simulink library "vmc"  (R2021b)
settings: Solver=VariableStepAuto  StartTime=0.0  StopTime=10.0  RelTol=1e-3
undefined symbols (not defined in the file or in its folder): AVMC_ACCDeltaTqIGain_X_kph, AVMC_ACCDeltaTqIGain_Y_mps2, AVMC_ACCDeltaTqIGainP2_X_kph, AVMC_ACCDeltaTqIGainP2_Y_mps2, AVMC_ACCDeltaTqPGain_X_kph, AVMC_ACCDeltaTqPGain_Y_kph, AVMC_ACCDeltaTqPGainP2_X_kph, AVMC_ACCDeltaTqPGainP2_Y_kph, AVMC_ACCLongSteadyCtrl_X_kph, AVMC_CCAccelCMD_X_kph, AVMC_CCAccelCMD_Y_kph, AVMC_CCDeltaTqIGain_X_kph, AVMC_CCDeltaTqIGain_Y_mps2, AVMC_CCDeltaTqPGain_X_kph, AVMC_CCDeltaTqPGain_Y_kph, AVMC_CCLongSteadyCtrl_X_kph, AVMC_DISCDeltaTqIGainP2_X_kph, AVMC_DISCDeltaTqIGainP2_Y_mps2, AVMC_ESCRegenOut_X_kph, AVMC_ESCRegenOut_Y_Deg, AVMC_ESCRegenOutEnSpd_X_Deg, AVMC_LatESCRegenOut_X_kph, AVMC_LatESCRegenOut_Y_Deg, AVMC_LongAccDeadZone_X_kph, AVMC_LongAccDeadZoneP2_X_kph, AVMC_LongAccFiltTs_X_Gps, AVMC_LongAccFiltTsP2_X_Gps, AVMC_MCPresBaseTq_X_bar, AVMC_MSAAccelCMD_X_kph, AVMC_MSAAccelCMD_Y_kph, AVMC_MSADeltaTqIGain_X_kph, AVMC_MSADeltaTqIGain_Y_mps2, AVMC_MSADeltaTqPGain_X_kph, AVMC_MSADeltaTqPGain_Y_kph, AVMC_MSALongSteadyCtrl_X_kph, AVMC_MSAPedalOvrd_X_kph, AVMC_MSASpdBand_X_kph, AVMC_OPDDisSlideRate_X_Deg, AVMC_RDCDetectTime_X_kph, AVMC_RDCDetectTime_Y_pct, AVMC_RDCEnSlideRate_X_Deg, AVMC_StESCYaw_X_kph, AVMC_StESCYaw_Y_Deg, AVMC_StESCYawCom_X_kph, AVMC_StESCYawCom_Y_Gps, AVMC_TMSpdBaseTq_X_rpm, C_TASK_10MS_S, C_TASK_5MS_S, DEG2RAD, Discrete, ENUM_ADASACCSTA_ACTIVE, ENUM_ADASACCSTA_OVERRIDE, ENUM_ADASACCSTA_STANDBY, ENUM_ADASMSASTA_ACTIVE, ENUM_ADASMSASTA_ERROR, ENUM_ADASMSASTA_OFF, ENUM_ADASMSASTA_OVERSPEED, ENUM_ADASMSASTA_STANDBY, ENUM_ADASMSASTA_UNDERSPEED, ENUM_ADASMSASTA_UNLIMIT ... (+254)
libraries: hcu_lib x57, simulink x49, ctrlSharedLib x6, simulink_extras x1
(part 4 of 9)

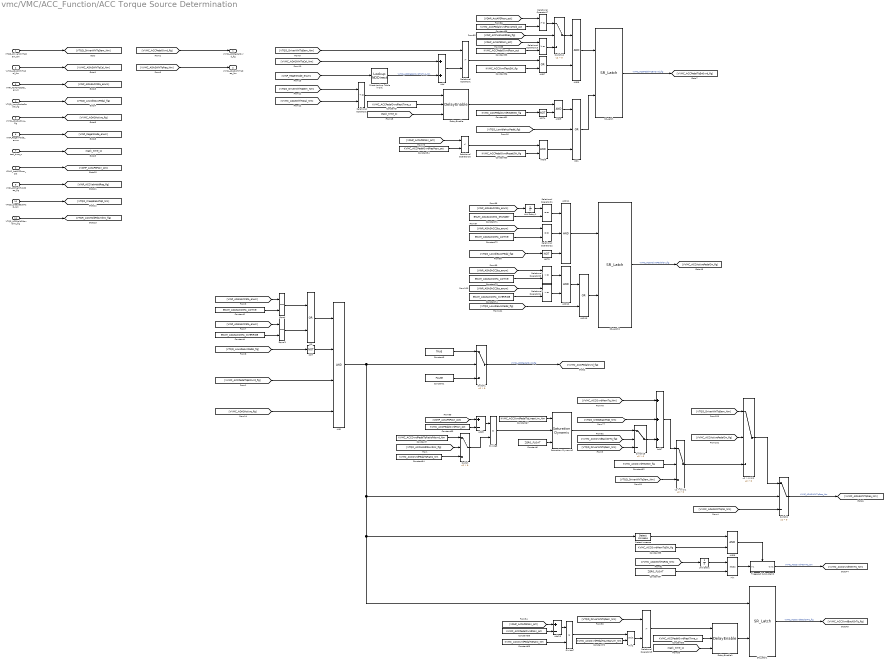
== system vmc/VMC/ACC_Function/ACC Torque Source Determination ==
  VTQD_DriverWhlTqDem_Nm : Inport
  VVMC_ADASWhlTqCal_Nm : Inport  Port=2
  VINP_ADASACCSta_enum : Inport  Port=3
  VTQD_LowIdleAccPedal_flg : Inport  Port=4
  VVMC_ADASActive_flg : Inport  Port=5
  VINP_RegenMode_enum : Inport  Port=6
  task_time_s : Inport  Port=7
  VDHP_ActAPSPosn_pct : Inport  Port=8
  VINP_ACCVehHoldReq_flg : Inport  Port=9
  VTQD_CreepBaseTqD_Nm : Inport  Port=10
  VTQR_ACCHoldPdovrdInc_flg : Inport  Port=11
  AND : Logic  Inputs=4  AllPortsSameDT=off  OutDataTypeStr=boolean
  AND11 : Logic  Inputs=3  AllPortsSameDT=off  OutDataTypeStr=boolean
  AND{5..6,8..9,12} (5 alike) : Logic  AllPortsSameDT=off  OutDataTypeStr=boolean
  AND13 : Logic  Operator=OR  AllPortsSameDT=off  OutDataTypeStr=boolean
  AND7 : Logic  Operator=OR  AllPortsSameDT=off  OutDataTypeStr=boolean
  Add : Sum
  Add13 : Sum  Inputs=+-
  Add7 : Sum  Inputs=+++
  Add8 : Sum  Inputs=+-
  Constant1 : Constant  Value=FALSE
  Constant2 : Constant  Value=ENUM_ADASACCSTA_ACTIVE
  Constant3 : Constant  Value=TRUE
  Constant4 : Constant  Value=ENUM_ADASACCSTA_OVERRIDE
  Constant5 : Constant  Value=KVMC_ACCPedalOvrdRestTime_s
  Constant53 : Constant  Value=KVMC_ACCPedalOvrdPosn_pct
  Constant54 : Constant  Value=KVMC_ACCPedalOvrdResPosn_pct
  Constant55 : Constant  Value=KVMC_ACCOvrdMemTqSW_flg
  Constant56 : Constant  Value=KVMC_ACCOvrdTestSW_flg
  Constant57 : Constant  Value=ZERO_FLOAT
  Constant58 : Constant  Value=KVMC_ACCPedalOvrdPosn4Hold_pct
  Constant6 : Constant  Value=ZERO_FLOAT
  Constant60 : Constant  Value=KVMC_ACCPedalOvrdResetSW_flg
  Constant61 : Constant  Value=KVMC_ACCPedalOvrdResetSW_flg
  Constant62 : Constant  Value=KVMC_ACCOvrdTestSW_flg
  Constant63 : Constant  Value=KVMC_ACCPedalOvrdPosn_pct
  Constant64 : Constant  Value=KVMC_ACCOvrdPedalTqRatio_Nm
  Constant66 : Constant  Value=KVMC_ACCPedalOvrdRestTime_s
  Constant67 : Constant  Value=KVMC_ACCOvrdPedalTqLinearLim_Nm
  Constant68 : Constant  Value=KVMC_ACCPedalOvrdPosn_pct
  Constant69 : Constant  Value=KVMC_ACCOvrdPedalTqRatio_Nm
  Constant7 : Constant  Value=KVMC_ACCOvrdPedalTqRatioPdovrd_Nm
  Constant70 : Constant  Value=KVMC_ACCOvrdPedalTqLinearLim_Nm
  Constant71 : Constant  Value=ENUM_ADASACCSTA_STANDBY
  Constant72 : Constant  Value=ENUM_ADASACCSTA_ACTIVE
  Constant73 : Constant  Value=ENUM_ADASACCSTA_ACTIVE
  Constant74 : Constant  Value=ENUM_ADASACCSTA_OVERRIDE
  DelayEnable : hcu_lib/Basic_Blocks/DelayEnable
  DelayEnable1 : hcu_lib/Basic_Blocks/DelayEnable
  Detect Increase : simulink/Logic and Bit Operations/Detect Increase  vinit=0.0  OutDataTypeStr=boolean
  Direct Lookup Table (n-D)1 : LookupNDDirect  NumberOfTableDimensions=1  Table=MVMC_ACCPedalOvrdTqHys_Y_Nm
  Divide5 : Product  Inputs=**
  Divide7 : Product  Inputs=**
  Equal : RelationalOperator  Operator===  OutDataTypeStr=boolean  RndMeth=Simplest
  Equal1 : RelationalOperator  Operator===  OutDataTypeStr=boolean  RndMeth=Simplest
  Min : MinMax  Function=max  Inputs=2
  Min2 : MinMax  Inputs=2
  NOT : Logic  Operator=NOT  AllPortsSameDT=off  OutDataTypeStr=boolean
  NOT4 : Logic  Operator=NOT  AllPortsSameDT=off  OutDataTypeStr=boolean
  NOT5 : Logic  Operator=NOT  AllPortsSameDT=off  OutDataTypeStr=boolean
  OR : Logic  Operator=OR  AllPortsSameDT=off  OutDataTypeStr=boolean
  OR1 : Logic  Operator=OR  Inputs=3  AllPortsSameDT=off  OutDataTypeStr=boolean
  Relational Operator1 : RelationalOperator  Operator=>  OutDataTypeStr=boolean  RndMeth=Simplest
  Relational Operator15 : RelationalOperator  OutDataTypeStr=boolean  RndMeth=Simplest
  Relational Operator16 : RelationalOperator  Operator=<  OutDataTypeStr=boolean  RndMeth=Simplest
  Relational Operator17 : RelationalOperator  OutDataTypeStr=boolean  RndMeth=Simplest
  Relational Operator19 : RelationalOperator  Operator=>  OutDataTypeStr=boolean  RndMeth=Simplest
  Relational Operator2 : RelationalOperator  Operator=<=  OutDataTypeStr=boolean  RndMeth=Simplest
  Relational Operator21 : RelationalOperator  Operator===  OutDataTypeStr=boolean  RndMeth=Simplest
  Relational Operator22 : RelationalOperator  Operator===  OutDataTypeStr=boolean  RndMeth=Simplest
  Relational Operator23 : RelationalOperator  Operator=~=  OutDataTypeStr=boolean  RndMeth=Simplest
  Relational Operator24 : RelationalOperator  Operator=~=  OutDataTypeStr=boolean  RndMeth=Simplest
  SR_Latch : hcu_lib/Basic_Blocks/SR_Latch
  SR_Latch1 : hcu_lib/Basic_Blocks/SR_Latch
  SR_Latch2 : hcu_lib/Basic_Blocks/SR_Latch
  Saturation Dynamic2 : simulink/Discontinuities/Saturation Dynamic  OutMin=[]  OutMax=[]  OutDataTypeStr=Inherit: Same as second input  OutDataType=fixdt(1, 16)  OutScaling=2^-10  DoSatur=off
  Switch{,1..2,12,15} (5 alike) : Switch  Criteria=u2 > Threshold
  Triggered Subsystem2 : Subsystem  TreatAsAtomicUnit=on
  Unit Delay : UnitDelay  SampleTime=-1  HasFrameUpgradeWarning=on
  Unit Delay1 : UnitDelay  SampleTime=-1  HasFrameUpgradeWarning=on
  u2 > 0 (1)1 : Switch  Criteria=u2 > Threshold
  u2 > 0 (1)2 : Switch  Criteria=u2 > Threshold
  VVMC_ACCPedalOvrd_flg : Outport
  VVMC_ADASWhlTqReq_Nm : Outport  Port=2
  wires:
  VTQD_DriverWhlTqDem_Nm/1 -> [VTQD_DriverWhlTqDem_Nm]
  VVMC_ADASWhlTqCal_Nm/1 -> [VVMC_ADASWhlTqCal_Nm]
  [VVMC_ACCPedalOvrd_flg] -> VVMC_ACCPedalOvrd_flg/1
  [VVMC_ADASWhlTqReq_Nm] -> VVMC_ADASWhlTqReq_Nm/1
  Switch2/1 -> [VVMC_ADASWhlTqReq_Nm]  "VVMC_ADASWhlTqReq_Nm"
  [VVMC_ADASWhlTqCal_Nm] -> Switch2/3
  Constant1/1 -> Switch1/3
  Constant3/1 -> Switch1/1
  Switch1/1 -> [VVMC_ACCPedalOvrd_flg]  "VVMC_ACCPedalOvrd_flg"
  Constant4/1 -> Equal1/2
  [VINP_ADASACCSta_enum] -> Equal/1
  Equal1/1 -> OR/2
  Equal/1 -> OR/1
  [VINP_ADASACCSta_enum] -> Equal1/1
  Constant2/1 -> Equal/2
  OR/1 -> AND/1
  VINP_ADASACCSta_enum/1 -> [VINP_ADASACCSta_enum]
  VTQD_LowIdleAccPedal_flg/1 -> [VTQD_LowIdleAccPedal_flg]
  NOT/1 -> AND/2
  [VTQD_LowIdleAccPedal_flg] -> NOT/1
  VVMC_ADASActive_flg/1 -> [VVMC_ADASActive_flg]
  VINP_RegenMode_enum/1 -> [VINP_RegenMode_enum]
  [VINP_RegenMode_enum] -> Direct Lookup Table (n-D)1/1
  Direct Lookup Table (n-D)1/1 -> Add/2  "VVMC_ACCPedalOvrdTqHys_Nm"
  [VVMC_ADASWhlTqCal_Nm] -> Relational Operator2/2
  [VVMC_ADASWhlTqCal_Nm] -> Add/1
  [VTQD_DriverWhlTqDem_Nm] -> Relational Operator2/1
  Add/1 -> Relational Operator1/2
  SR_Latch/1 -> [VVMC_ACCPedalTqEnOvrd_flg]  "VVMC_ACCPedalTqEnOvrd_flg"
  [VTQD_DriverWhlTqDem_Nm] -> Relational Operator1/1
  [VVMC_ADASActive_flg] -> AND/4
  [VVMC_ACCPedalTqEnOvrd_flg] -> AND/3
  Relational Operator2/1 -> DelayEnable/1
  [task_time_s] -> DelayEnable/3
  Constant5/1 -> DelayEnable/2
  task_time_s/1 -> [task_time_s]
  OR1/1 -> SR_Latch/2
  [VTQD_LowIdleAccPedal_flg] -> OR1/2
  Switch12/1 -> AND5/1
  AND7/1 -> AND5/2
  Constant56/1 -> AND7/2
  [VDHP_ActAPSPosn_pct] -> Relational Operator17/1
  Relational Operator1/1 -> AND7/1
  Constant53/1 -> Relational Operator15/2
  Relational Operator15/1 -> Switch12/3
  [VDHP_ActAPSPosn_pct] -> Relational Operator15/1
  Relational Operator17/1 -> Switch12/1
  Constant58/1 -> Relational Operator17/2
  [VINP_ACCVehHoldReq_flg] -> Switch12/2
  AND5/1 -> SR_Latch/1
  [VDHP_ActAPSPosn_pct] -> Relational Operator16/1
  DelayEnable/1 -> AND9/1
  Constant61/1 -> NOT4/1
  AND9/1 -> OR1/1
  Constant60/1 -> AND8/2
  NOT4/1 -> AND9/2
  Constant54/1 -> Relational Operator16/2
  Relational Operator16/1 -> AND8/1
  AND8/1 -> OR1/3
  Switch15/1 -> Add7/3
  Add7/1 -> u2 > 0 (1)1/1
  [VTQD_CreepBaseTqD_Nm] -> Add7/2
  [VTQD_DriverWhlTqDem_Nm] -> Switch15/3
  Divide5/1 -> Saturation Dynamic2/2
  Saturation Dynamic2/1 -> Switch15/1
  Constant63/1 -> Add8/2
  u2 > 0 (1)2/1 -> Switch2/1
  [VVMC_ACCOvrdBackDrTq_flg] -> Switch15/2
  Add8/1 -> Divide5/1
  u2 > 0 (1)1/1 -> u2 > 0 (1)2/3
  [VDHP_ActAPSPosn_pct] -> Add8/1
  [VVMC_ACCActivePedalOn_flg] -> u2 > 0 (1)2/2
  Switch/1 -> Divide5/2
  [VTQD_DriverWhlTqDem_Nm] -> u2 > 0 (1)1/3
  Constant62/1 -> u2 > 0 (1)1/2
  [VTQD_DriverWhlTqDem_Nm] -> u2 > 0 (1)2/1
  Min/1 -> Triggered Subsystem2/1(In1)
  AND6/1 -> Triggered Subsystem2/Trigger
  AND/1 -> Switch1/2, Switch2/2, Detect Increase/1, SR_Latch1/1
  Detect Increase/1 -> AND6/1
  Triggered Subsystem2/1(Out1) -> [VVMC_ACCOvrdMemTq_Nm]  "VVMC_ACCOvrdMemTq_Nm"
  [task_time_s] -> DelayEnable1/3
  [VVMC_ADASWhlTqReq_Nm] -> Unit Delay/1
  Unit Delay/1 -> Min/1
  Constant57/1 -> Min/2
  SR_Latch1/1 -> [VVMC_ACCOvrdBackDrTq_flg]  "VVMC_ACCOvrdBackDrTq_flg"
  Constant55/1 -> AND6/2
  [VTQD_DriverWhlTqDem_Nm] -> Relational Operator19/1
  DelayEnable1/1 -> SR_Latch1/2
  Constant66/1 -> DelayEnable1/2
  Constant70/1 -> Min2/2
  Min2/1 -> Relational Operator19/2
  Add13/1 -> Divide7/1
  Relational Operator19/1 -> DelayEnable1/1
  Divide7/1 -> Min2/1
  [VDHP_ActAPSPosn_pct] -> Add13/1
  Constant69/1 -> Divide7/2
  Constant68/1 -> Add13/2
  Relational Operator24/1 -> AND12/2
  AND12/1 -> AND13/1
  Constant74/1 -> Relational Operator24/2
  NOT5/1 -> AND11/3
  Constant71/1 -> Relational Operator21/2
  AND13/1 -> SR_Latch2/2
  Constant72/1 -> Relational Operator22/2
  Relational Operator23/1 -> AND12/1
  Unit Delay1/1 -> Relational Operator21/1
  AND11/1 -> SR_Latch2/1
  Relational Operator22/1 -> AND11/2
  SR_Latch2/1 -> [VVMC_ACCActivePedalOn_flg]  "VVMC_ACCActivePedalOn_flg"
  [VINP_ADASACCSta_enum] -> Relational Operator24/1
  Constant73/1 -> Relational Operator23/2
  [VINP_ADASACCSta_enum] -> Relational Operator23/1
  Relational Operator21/1 -> AND11/1
  [VINP_ADASACCSta_enum] -> Relational Operator22/1
  [VTQD_LowIdleAccPedal_flg] -> NOT5/1
  [VTQD_LowIdleAccPedal_flg] -> AND13/2
  [VINP_ADASACCSta_enum] -> Unit Delay1/1
  VDHP_ActAPSPosn_pct/1 -> [VDHP_ActAPSPosn_pct]
  VINP_ACCVehHoldReq_flg/1 -> [VINP_ACCVehHoldReq_flg]
  VTQD_CreepBaseTqD_Nm/1 -> [VTQD_CreepBaseTqD_Nm]
  Constant67/1 -> Saturation Dynamic2/1
  Constant6/1 -> Saturation Dynamic2/3
  [VVMC_ACCOvrdMemTq_Nm] -> Add7/1
  VTQR_ACCHoldPdovrdInc_flg/1 -> [VTQR_ACCHoldPdovrdInc_flg]
  [VTQR_ACCHoldPdovrdInc_flg] -> Switch/2
  Constant64/1 -> Switch/3
  Constant7/1 -> Switch/1

== system vmc/VMC/ACC_Function/Hand Shaking ==
  VINP_ADASACCSta_enum : Inport
  VVMC_ACCCtrlAllow_flg : Inport  Port=2
  Constant1 : Constant  Value=TRUE
  Constant2 : Constant  Value=ENUM_ADASACCSTA_ACTIVE
  Constant3 : Constant  Value=FALSE
  Constant4 : Constant  Value=ENUM_ADASACCSTA_OVERRIDE
  Constant5 : Constant  Value=TRUE
  Constant6 : Constant  Value=FALSE
  Logical Operator : Logic  AllPortsSameDT=off  OutDataTypeStr=boolean
  OR : Logic  Operator=OR  AllPortsSameDT=off  OutDataTypeStr=boolean
  Relational Operator1 : RelationalOperator  Operator===  OutDataTypeStr=boolean  RndMeth=Simplest
  Relational Operator2 : RelationalOperator  Operator===  OutDataTypeStr=boolean  RndMeth=Simplest
  Switch : Switch  Criteria=u2 > Threshold
  u2>0 : Switch  Criteria=u2 > Threshold
  VVMC_ACCCtrlAvail_flg : Outport
  VVMC_ADASActive_flg : Outport  Port=2
  wires:
  [VVMC_ACCCtrlAvail_flg] -> VVMC_ACCCtrlAvail_flg/1
  VINP_ADASACCSta_enum/1 -> [VINP_ADASACCSta_enum]
  [VVMC_ADASActive_flg] -> VVMC_ADASActive_flg/1
  [VVMC_ACCCtrlAllow_flg] -> Switch/2, Logical Operator/2
  Switch/1 -> [VVMC_ACCCtrlAvail_flg]  "VVMC_ACCCtrlAvail_flg"
  Constant6/1 -> Switch/3
  Constant5/1 -> Switch/1
  VVMC_ACCCtrlAllow_flg/1 -> [VVMC_ACCCtrlAllow_flg]
  OR/1 -> Logical Operator/1
  Logical Operator/1 -> u2>0/2
  Constant1/1 -> u2>0/1
  u2>0/1 -> [VVMC_ADASActive_flg]  "VVMC_ADASActive_flg"
  Constant3/1 -> u2>0/3
  Relational Operator2/1 -> OR/2
  Relational Operator1/1 -> OR/1
  [VINP_ADASACCSta_enum] -> Relational Operator2/1
  Constant2/1 -> Relational Operator1/2
  [VINP_ADASACCSta_enum] -> Relational Operator1/1
  Constant4/1 -> Relational Operator2/2

== system vmc/VMC/ACC_ReqAccelControl/Triggered Subsystem4 ==
  In1 : Inport
  In2 : Inport  Port=2
  Trigger : TriggerPort  VariantControl=(inherit)
  Out1 : Outport
  Out2 : Outport  Port=2
  wires:
  In2/1 -> Out2/1
  In1/1 -> Out1/1

== system vmc/VMC/ACC_ReqAccelControl/Triggered Subsystem5 ==
  In1 : Inport
  Trigger : TriggerPort  VariantControl=(inherit)
  Out1 : Outport
  wires:
  In1/1 -> Out1/1

== system vmc/VMC/APS function/CAAS HandShake ==
  VINP_VehSpeed_kph : Inport
  VVMC_ADASActive_flg : Inport  Port=2
  VVMC_CruzActive_flg : Inport  Port=3
  task_time_s : Inport  Port=4
  VINP_CAASVMCReqA_flg : Inport  Port=5
  AND : Logic  Inputs=3  AllPortsSameDT=off  OutDataTypeStr=boolean
  AND1 : Logic  AllPortsSameDT=off  OutDataTypeStr=boolean
  Constant1 : Constant  Value=KVMC_CAASCtrlAllowTime_s
  Constant11 : Constant  Value=KVMC_CAASEnVehSpd_kph
  Constant2 : Constant  Value=KVMC_CAASVMCReqA_flg_ovrdflg
  Constant3 : Constant  Value=KVMC_CAASVMCReqA_flg_ovrdval
  DelayEnable : hcu_lib/Basic_Blocks/DelayEnable
  NOT : Logic  Operator=NOT  AllPortsSameDT=off  OutDataTypeStr=boolean
  NOT1 : Logic  Operator=NOT  AllPortsSameDT=off  OutDataTypeStr=boolean
  Relational Operator : RelationalOperator  Operator=<=  OutDataTypeStr=boolean  RndMeth=Simplest
  Switch : Switch  Criteria=u2 > Threshold
  VVMC_CAASCtrlAvail_flg : Outport
  VVMC_CAASActive_flg : Outport  Port=2
  wires:
  Relational Operator/1 -> AND/1
  VVMC_ADASActive_flg/1 -> [VVMC_ADASActive_flg]
  VINP_VehSpeed_kph/1 -> [VINP_VehSpeed_kph]
  AND/1 -> DelayEnable/1
  Constant1/1 -> DelayEnable/2
  task_time_s/1 -> [task_time_s]
  [VINP_VehSpeed_kph] -> Relational Operator/1
  [VVMC_CruzActive_flg] -> NOT1/1
  VVMC_CruzActive_flg/1 -> [VVMC_CruzActive_flg]
  Constant11/1 -> Relational Operator/2
  DelayEnable/1 -> [VVMC_CAASCtrlAvail_flg]  "VVMC_CAASCtrlAvail_flg"
  [task_time_s] -> DelayEnable/3
  NOT1/1 -> AND/3
  NOT/1 -> AND/2
  [VVMC_ADASActive_flg] -> NOT/1
  [VVMC_CAASCtrlAvail_flg] -> VVMC_CAASCtrlAvail_flg/1
  [VVMC_CAASCtrlAvail_flg] -> AND1/1
  VINP_CAASVMCReqA_flg/1 -> [VINP_CAASVMCReqA_flg]
  AND1/1 -> [VVMC_CAASActive_flg]  "VVMC_CAASActive_flg"
  [VVMC_CAASActive_flg] -> VVMC_CAASActive_flg/1
  [VINP_CAASVMCReqA_flg] -> Switch/3
  Switch/1 -> AND1/2
  Constant3/1 -> Switch/1
  Constant2/1 -> Switch/2

== system vmc/VMC/APS function/Command Determination ==
  VVMC_APSActive_flg : Inport
  VINP_APSStaSys_enum : Inport  Port=2
  VINP_APSShiftPosnReq_enum : Inport  Port=3
  VINP_APSSpeedCMD_kph : Inport  Port=4
  AND : Logic  AllPortsSameDT=off  OutDataTypeStr=boolean
  Constant : Constant  Value=ENUM_APSSYSTEMSTA_ACTIVE
  Constant1 : Constant  Value=ENUM_APSSYSTEMSTA_REMOTEACTIVE
  Constant2 : Constant  Value=ZERO_FLOAT
  Constant3 : Constant  Value=ENUM_APSSHIFTPOSNREQ_PARK
  Equal : RelationalOperator  Operator===  OutDataTypeStr=boolean  RndMeth=Simplest
  Equal1 : RelationalOperator  Operator===  OutDataTypeStr=boolean  RndMeth=Simplest
  OR : Logic  Operator=OR  AllPortsSameDT=off  OutDataTypeStr=boolean
  Switch : Switch  Criteria=u2 > Threshold
  Switch1 : Switch  Criteria=u2 > Threshold
  VVMC_APSSpeedCMD_kph : Outport
  VVMC_APSShiftPosnReq_enum : Outport  Port=2
  wires:
  [VVMC_APSEnCMD_flg] -> Switch1/2
  [VINP_APSShiftPosnReq_enum] -> Switch1/1
  Constant3/1 -> Switch1/3
  Switch1/1 -> VVMC_APSShiftPosnReq_enum/1  "VVMC_APSShiftPosnReq_enum"
  Switch/1 -> VVMC_APSSpeedCMD_kph/1  "VVMC_APSSpeedCMD_kph"
  Constant2/1 -> Switch/3
  [VINP_APSSpeedCMD_kph] -> Switch/1
  [VVMC_APSEnCMD_flg] -> Switch/2
  AND/1 -> [VVMC_APSEnCMD_flg]  "VVMC_APSEnCMD_flg"
  OR/1 -> AND/2
  [VVMC_APSActive_flg] -> AND/1
  Equal1/1 -> OR/2
  Equal/1 -> OR/1
  [VINP_APSStaSys_enum] -> Equal1/1
  Constant1/1 -> Equal1/2
  Constant/1 -> Equal/2
  [VINP_APSStaSys_enum] -> Equal/1
  VINP_APSSpeedCMD_kph/1 -> [VINP_APSSpeedCMD_kph]
  VINP_APSShiftPosnReq_enum/1 -> [VINP_APSShiftPosnReq_enum]
  VINP_APSStaSys_enum/1 -> [VINP_APSStaSys_enum]
  VVMC_APSActive_flg/1 -> [VVMC_APSActive_flg]

== system vmc/VMC/APS function/Hand Shake ==
  task_time_s : Inport
  VTQD_ExternalTqAllow_flg : Inport  Port=2
  VTQD_ExtShiftAllow_flg : Inport  Port=3
  VINP_APSVMCReqA_flg : Inport  Port=4
  VINP_APSStaSys_enum : Inport  Port=5
  VTQD_ExtDoorAllow_flg : Inport  Port=6
  AND : Logic  Inputs=3  AllPortsSameDT=off  OutDataTypeStr=boolean
  AND1 : Logic  Inputs=3  AllPortsSameDT=off  OutDataTypeStr=boolean
  AND2 : Logic  AllPortsSameDT=off  OutDataTypeStr=boolean
  Constant : Constant  Value=KVMC_ExternalTqAllowTime_s
  Constant1 : Constant  Value=KVMC_ExternalShiftAllowTime_s
  Constant2 : Constant  Value=ENUM_APSSYSTEMSTA_ACTIVE
  Constant3 : Constant  Value=ENUM_APSSYSTEMSTA_REMOTEACTIVE
  Constant4 : Constant  Value=KVMC_ExternalDoorAllowTime_s
  Delay : Delay  DelayLength=1
  Delay1 : Delay  DelayLength=1
  DelayEnable : hcu_lib/Basic_Blocks/DelayEnable
  DelayEnable1 : hcu_lib/Basic_Blocks/DelayEnable
  DelayEnable2 : hcu_lib/Basic_Blocks/DelayEnable
  Detect Decrease : simulink/Logic and Bit Operations/Detect Decrease  vinit=0.0  OutDataTypeStr=boolean
  Equal : RelationalOperator  Operator===  OutDataTypeStr=boolean  RndMeth=Simplest
  Equal1 : RelationalOperator  Operator===  OutDataTypeStr=boolean  RndMeth=Simplest
  NOT : Logic  Operator=NOT  AllPortsSameDT=off  OutDataTypeStr=boolean
  OR : Logic  Operator=OR  AllPortsSameDT=off  OutDataTypeStr=boolean
  SR_Latch : hcu_lib/Basic_Blocks/SR_Latch
  VVMC_APSCtrlAvail_flg : Outport
  VVMC_APSActive_flg : Outport  Port=2
  wires:
  VINP_APSVMCReqA_flg/1 -> [VINP_APSVMCReqA_flg]
  VTQD_ExtShiftAllow_flg/1 -> [VTQD_ExtShiftAllow_flg]
  [task_time_s] -> DelayEnable1/3
  Constant1/1 -> DelayEnable1/2
  DelayEnable1/1 -> [VVMC_APSShiftCtrlAllow_flg]  "VVMC_APSShiftCtrlAllow_flg"
  [VTQD_ExtShiftAllow_flg] -> DelayEnable1/1
  [VTQD_ExternalTqAllow_flg] -> DelayEnable/1
  VTQD_ExternalTqAllow_flg/1 -> [VTQD_ExternalTqAllow_flg]
  task_time_s/1 -> [task_time_s]
  DelayEnable/1 -> [VVMC_APSTqCtrlAllow_flg]  "VVMC_APSTqCtrlAllow_flg"
  Constant/1 -> DelayEnable/2
  [task_time_s] -> DelayEnable/3
  Constant2/1 -> Equal/2
  [VINP_APSStaSys_enum] -> Equal/1
  Equal/1 -> OR/1
  OR/1 -> AND1/3
  [VINP_APSVMCReqA_flg] -> AND1/1
  Constant3/1 -> Equal1/2
  Equal1/1 -> OR/2
  [VINP_APSStaSys_enum] -> Equal1/1
  [VVMC_APSCtrlAvail_flg] -> AND1/2
  AND1/1 -> [VVMC_APSActive_flg], VVMC_APSActive_flg/1  "VVMC_APSActive_flg"
  VINP_APSStaSys_enum/1 -> [VINP_APSStaSys_enum]
  VTQD_ExtDoorAllow_flg/1 -> [VTQD_ExtDoorAllow_flg]
  Constant4/1 -> DelayEnable2/2
  DelayEnable2/1 -> [VVMC_APSDoorCtrlAllow_flg]  "VVMC_APSDoorCtrlAllow_flg"
  [task_time_s] -> DelayEnable2/3
  [VTQD_ExtDoorAllow_flg] -> DelayEnable2/1
  [VVMC_APSActive_flg] -> Delay1/1
  SR_Latch/1 -> AND/3
  [VVMC_APSActive_flg] -> Delay/1
  Delay/1 -> NOT/1
  NOT/1 -> AND2/2
  AND2/1 -> SR_Latch/1
  Delay1/1 -> Detect Decrease/1
  Detect Decrease/1 -> SR_Latch/2
  [VVMC_APSDoorCtrlAllow_flg] -> AND2/1
  AND/1 -> [VVMC_APSCtrlAvail_flg], VVMC_APSCtrlAvail_flg/1  "VVMC_APSCtrlAvail_flg"
  [VVMC_APSTqCtrlAllow_flg] -> AND/1
  [VVMC_APSShiftCtrlAllow_flg] -> AND/2

== system vmc/VMC/APS function/Signal Rounting ==
  VINP_SCPSystemMode_enum : Inport
  BTQD_outputs : Inport  Port=2  OutDataTypeStr=Bus: BTQD_outputs
  VVMC_APSActive_flg : Inport  Port=3
  VVMC_ADASActive_flg : Inport  Port=4
  BINP_APM_outputs : Inport  Port=5
  VTQD_GearActualPosn_enum : Inport  Port=6
  VVMC_CAASActive_flg : Inport  Port=7
  VVMC_SetACCDisableAPS_flg : Inport  Port=8
  Bus Selector1 : BusSelector  OutputSignals=VTQD_APSStaSys_enum
  Bus Selector2 : BusSelector  OutputSignals=VINP_APSStaSystem_enum
  Bus Selector3 : BusSelector  OutputSignals=VTQD_APSDecReqA_flg
  Bus Selector4 : BusSelector  OutputSignals=VINP_APSDecReqA_flg
  Bus Selector5 : BusSelector  OutputSignals=VINP_APSDecReq_mps2
  Bus Selector6 : BusSelector  OutputSignals=VINP_APSReq_enum
  Bus Selector7 : BusSelector  OutputSignals=VTQD_APSDecReq_mps2
  Bus Selector9 : BusSelector  OutputSignals=VTQD_APSReq_enum
  Signal Determination VINP_APSDecReqAtest_flg : Subsystem
  Signal Determination VINP_APSDecReqtest_mps2 : Subsystem
  Signal Determination VINP_APSReqtest_enum : Subsystem
  Signal Determination VINP_APSStaSystemtest_enum : Subsystem
  Switch{,1..3} (4 alike) : Switch  Criteria=u2 > Threshold
  VVMC_APSStaSys_enum : Outport
  VVMC_APSDecReqA_flg : Outport  Port=2
  VVMC_APSDecReq_mps2 : Outport  Port=3
  VVMC_APSReq_enum : Outport  Port=4
  wires:
  [VINP_SCPSystemMode_enum] -> Signal Determination VINP_APSDecReqtest_mps2/3(VINP_SCPSystemMode_enum)
  Signal Determination VINP_APSDecReqAtest_flg/1(SignalOutp) -> VVMC_APSDecReqA_flg/1  "VVMC_APSDecReqA_flg"
  Signal Determination VINP_APSReqtest_enum/1(SignalOutp) -> VVMC_APSReq_enum/1  "VVMC_APSReq_enum"
  [VINP_SCPSystemMode_enum] -> Signal Determination VINP_APSReqtest_enum/3(VINP_SCPSystemMode_enum)
  Signal Determination VINP_APSStaSystemtest_enum/1(SignalOutp) -> VVMC_APSStaSys_enum/1  "VVMC_APSStaSys_enum"
  [VINP_SCPSystemMode_enum] -> Signal Determination VINP_APSDecReqAtest_flg/3(VINP_SCPSystemMode_enum)
  Signal Determination VINP_APSDecReqtest_mps2/1(SignalOutp) -> VVMC_APSDecReq_mps2/1  "VVMC_APSDecReq_mps2"
  BTQD_outputs/1 -> [BTQD_outputs]
  VINP_SCPSystemMode_enum/1 -> [VINP_SCPSystemMode_enum]
  VVMC_APSActive_flg/1 -> [VVMC_APSActive_flg]
  VVMC_ADASActive_flg/1 -> [VVMC_ADASActive_flg]
  [VVMC_APSActive_flg] -> Signal Determination VINP_APSStaSystemtest_enum/4(VVMC_APSActive_flg)
  [VVMC_ADASActive_flg] -> Signal Determination VINP_APSStaSystemtest_enum/5(VVMC_ADASActive_flg)
  [VVMC_APSActive_flg] -> Signal Determination VINP_APSDecReqAtest_flg/4(VVMC_APSActive_flg)
  [VVMC_ADASActive_flg] -> Signal Determination VINP_APSDecReqAtest_flg/5(VVMC_ADASActive_flg)
  [VVMC_APSActive_flg] -> Signal Determination VINP_APSDecReqtest_mps2/4(VVMC_APSActive_flg)
  [VVMC_ADASActive_flg] -> Signal Determination VINP_APSDecReqtest_mps2/5(VVMC_ADASActive_flg)
  [VVMC_APSActive_flg] -> Signal Determination VINP_APSReqtest_enum/4(VVMC_APSActive_flg)
  [VVMC_ADASActive_flg] -> Signal Determination VINP_APSReqtest_enum/5(VVMC_ADASActive_flg)
  VTQD_GearActualPosn_enum/1 -> [VTQD_GearActualPosn_enum]
  BINP_APM_outputs/1 -> [BINP_APM_outputs]
  [VTQD_GearActualPosn_enum] -> Signal Determination VINP_APSStaSystemtest_enum/6(VTQD_GearActualPosn_enum)
  [VINP_SCPSystemMode_enum] -> Signal Determination VINP_APSStaSystemtest_enum/3(VINP_SCPSystemMode_enum)
  Bus Selector2/1 -> Switch/1, Signal Determination VINP_APSStaSystemtest_enum/1(SignalInput1)  "<VINP_APSStaSystem_enum>"
  [BINP_APM_outputs] -> Bus Selector2/1
  Bus Selector4/1 -> Switch1/1, Signal Determination VINP_APSDecReqAtest_flg/1(SignalInput1)  "<VINP_APSDecReqA_flg>"
  [BINP_APM_outputs] -> Bus Selector4/1
  Bus Selector5/1 -> Switch2/1, Signal Determination VINP_APSDecReqtest_mps2/1(SignalInput1)  "<VINP_APSDecReq_mps2>"
  [BINP_APM_outputs] -> Bus Selector5/1
  Bus Selector6/1 -> Switch3/1, Signal Determination VINP_APSReqtest_enum/1(SignalInput1)  "<VINP_APSReq_enum>"
  [BINP_APM_outputs] -> Bus Selector6/1
  VVMC_CAASActive_flg/1 -> [VVMC_CAASActive_flg]
  [VVMC_CAASActive_flg] -> Signal Determination VINP_APSStaSystemtest_enum/7(VVMC_CAASActive_flg)
  [VVMC_CAASActive_flg] -> Signal Determination VINP_APSDecReqAtest_flg/6(VVMC_CAASActive_flg)
  [VVMC_CAASActive_flg] -> Signal Determination VINP_APSDecReqtest_mps2/6(VVMC_CAASActive_flg)
  [VVMC_CAASActive_flg] -> Signal Determination VINP_APSReqtest_enum/6(VVMC_CAASActive_flg)
  [VVMC_SetACCDisableAPS_flg] -> Switch1/2
  Bus Selector9/1 -> Switch3/3  "<VTQD_APSReq_enum>"
  [VVMC_SetACCDisableAPS_flg] -> Switch/2
  [VVMC_SetACCDisableAPS_flg] -> Switch2/2
  Bus Selector1/1 -> Switch/3  "<VTQD_APSStaSys_enum>"
  [BTQD_outputs] -> Bus Selector1/1
  Bus Selector3/1 -> Switch1/3  "<VTQD_APSDecReqA_flg>"
  [BTQD_outputs] -> Bus Selector3/1
  [BTQD_outputs] -> Bus Selector7/1
  [BTQD_outputs] -> Bus Selector9/1
  Bus Selector7/1 -> Switch2/3  "<VTQD_APSDecReq_mps2>"
  [VVMC_SetACCDisableAPS_flg] -> Switch3/2
  Switch3/1 -> Signal Determination VINP_APSReqtest_enum/2(SignalInput2)
  Switch2/1 -> Signal Determination VINP_APSDecReqtest_mps2/2(SignalInput2)
  Switch1/1 -> Signal Determination VINP_APSDecReqAtest_flg/2(SignalInput2)
  Switch/1 -> Signal Determination VINP_APSStaSystemtest_enum/2(SignalInput2)
  VVMC_SetACCDisableAPS_flg/1 -> [VVMC_SetACCDisableAPS_flg]

== system vmc/VMC/CruiseControlFunction/CCActiveDetermination ==
  VINP_ZoneSpdCrlMode_enum : Inport
  VTQD_ExternalTqAllow_flg : Inport  Port=2
  VINP_SWCSetdownSta_flg : Inport  Port=3
  VINP_SWCResUpSta_flg : Inport  Port=4
  VINP_VehSpeed_kph : Inport  Port=5
  VINP_SetSpd_kph : Inport  Port=6
  VINP_BrakeSWGPIO_flg : Inport  Port=7
  VINP_SWCCANCELSta_flg : Inport  Port=8
  VINP_BrkSwSta_flg : Inport  Port=9
  VVMC_CCPedalOvrd_flg : Inport  Port=10
  VTQD_GearActualPosn_enum : Inport  Port=11
  VINP_BrkPedalPos_pct : Inport  Port=12
  VTQD_ExtDoorAllow_flg : Inport  Port=13
  VVMC_CalMeterSpeed_kph : Inport  Port=14
  Chart : Stateflow chart  TreatAsAtomicUnit=on
  Constant : Constant  Value=KVMC_CCActiveMetSpdHi_kph
  Constant1 : Constant  Value=KVMC_CCActiveMetSpdLo_kph
  Constant2 : Constant  Value=KVMC_CCMSASpdWar_kph
  Constant3 : Constant  Value=KVMC_CCDisBrkPos_pct
  Constant4 : Constant  Value=KVMC_CCModeEnSpd_kph
  Data Type Conversion3 : DataTypeConversion  OutDataTypeStr=uint8
  Delay : Delay  DelayLength=1
  Detect Decrease : simulink/Logic and Bit Operations/Detect Decrease  vinit=0.0  OutDataTypeStr=boolean
  Detect Decrease1 : simulink/Logic and Bit Operations/Detect Decrease  vinit=0.0  OutDataTypeStr=boolean
  Detect Decrease2 : simulink/Logic and Bit Operations/Detect Decrease  vinit=0.0  OutDataTypeStr=boolean
  VVMC_CCCtrlSta_enum : Outport
  VVMC_CCSpdWar_flg : Outport  Port=2
  VVMC_CruzActive_flg : Outport  Port=3
  wires:
  Delay/1 -> Chart/13(VVMC_CCPedalOvrd_flg)
  VVMC_CCPedalOvrd_flg/1 -> [VVMC_CCPedalOvrd_flg]
  [VVMC_CCPedalOvrd_flg] -> Delay/1
  [VINP_BrkSwSta_flg] -> Chart/11(VINP_BrkSwSta_flg)
  Chart/1(VVMC_CCCtrlSta_enum) -> [VVMC_CCCtrlSta_enum]  "VVMC_CCCtrlSta_enum"
  Chart/3(VVMC_CruzActive_flg) -> [VVMC_CruzActive_flg]  "VVMC_CruzActive_flg"
  Chart/2(VVMC_CCSpdWar_flg) -> [VVMC_CCSpdWar_flg]  "VVMC_CCSpdWar_flg"
  Detect Decrease2/1 -> Chart/12(VVMC_DetectSWCResUp_flg)  "VVMC_DetectSWCResUp_flg"
  Detect Decrease1/1 -> Chart/10(VVMC_DetectSWCCANCEL_flg)  "VVMC_DetectSWCCANCEL_flg"
  Detect Decrease/1 -> Chart/3(VVMC_DetectSWCSetDown_flg)  "VVMC_DetectSWCSetDown_flg"
  [VVMC_CruzActive_flg] -> VVMC_CruzActive_flg/1
  [VVMC_CCSpdWar_flg] -> VVMC_CCSpdWar_flg/1
  [VVMC_CCCtrlSta_enum] -> VVMC_CCCtrlSta_enum/1
  VINP_BrkSwSta_flg/1 -> [VINP_BrkSwSta_flg]
  VINP_SWCCANCELSta_flg/1 -> [VINP_SWCCANCELSta_flg]
  VINP_BrakeSWGPIO_flg/1 -> [VINP_BrakeSWGPIO_flg]
  VINP_SetSpd_kph/1 -> [VINP_SetSpd_kph]
  VINP_VehSpeed_kph/1 -> [VINP_VehSpeed_kph]
  VINP_SWCResUpSta_flg/1 -> [VINP_SWCResUpSta_flg]
  VINP_SWCSetdownSta_flg/1 -> [VINP_SWCSetdownSta_flg]
  VTQD_ExternalTqAllow_flg/1 -> [VTQD_ExternalTqAllow_flg]
  VINP_ZoneSpdCrlMode_enum/1 -> [VINP_ZoneSpdCrlMode_enum]
  [VINP_SWCResUpSta_flg] -> Detect Decrease2/1
  [VINP_SWCCANCELSta_flg] -> Detect Decrease1/1
  [VINP_BrakeSWGPIO_flg] -> Chart/9(VINP_BrakeSWGPIO_flg)
  [VINP_ZoneSpdCrlMode_enum] -> Chart/1(VINP_ZoneSpdCrlMode_enum)
  [VTQD_ExternalTqAllow_flg] -> Chart/2(VTQD_ExternalTqAllow_flg)
  Constant2/1 -> Chart/8(KVMC_CCMSASpdWar_kph)
  [VINP_SetSpd_kph] -> Data Type Conversion3/1
  [VINP_SWCSetdownSta_flg] -> Detect Decrease/1
  Constant1/1 -> Chart/6(KVMC_CCActiveMetSpdLo_kph)
  [VINP_VehSpeed_kph] -> Chart/5(VINP_VehSpeed_kph)
  Constant/1 -> Chart/4(KVMC_CCActiveMetSpdHi_kph)
  [VTQD_GearActualPosn_enum] -> Chart/14(VTQD_GearActualPosn_enum)
  VTQD_GearActualPosn_enum/1 -> [VTQD_GearActualPosn_enum]
  Constant3/1 -> Chart/16(KVMC_CCDisBrkPos_pct)
  Constant4/1 -> Chart/17(KVMC_CCModeEnSpd_kph)
  VINP_BrkPedalPos_pct/1 -> [VINP_BrkPedalPos_pct]
  [VINP_BrkPedalPos_pct] -> Chart/15(VINP_BrkPedalPos_pct)
  Data Type Conversion3/1 -> Chart/7(VINP_SetSpd_kph)
  VTQD_ExtDoorAllow_flg/1 -> [VTQD_ExtDoorAllow_flg]
  [VTQD_ExtDoorAllow_flg] -> Chart/18(VTQD_ExtDoorAllow_flg)
  VVMC_CalMeterSpeed_kph/1 -> [VVMC_CalMeterSpeed_kph]
  [VVMC_CalMeterSpeed_kph] -> Chart/19(VVMC_CalMeterSpeed_kph)

== system vmc/VMC/CruiseControlFunction/CCDemandTorqueCalculation ==
  VINP_SetSpd_kph : Inport
  VINP_VehSpeed_kph : Inport  Port=2
  VVMC_CruzActive_flg : Inport  Port=3
  VTQD_DriverWhlTqDem_Nm : Inport  Port=4
  VVMC_LongAcc_Gps : Inport  Port=5
  VVMC_CCPedalOvrd_flg : Inport  Port=6
  VVMC_CalMeterSpeed_kph : Inport  Port=7
  Abs : Abs
  Add : Sum  Inputs=+-
  Add1 : Sum
  Add2 : Sum
  Add3 : Sum  Inputs=+-
  Add4 : Sum  Inputs=+-
  Add5 : Sum
  CC Mode Acceleration Determination : Lookup_n-D  BreakpointsForDimension1=AVMC_CCAccelCMD_Y_kph  BreakpointsForDimension2=AVMC_CCAccelCMD_X_kph  BreakpointsForDimension3=[5, 7]  Table=MVMC_CCAccelCMD_Z_mps2  ExtrapMethod=Clip  InternalRulePriority=Speed  RndMeth=Simplest  InputSameDT=on
      settings: InputPortMap=u0,u1
  Constant : Constant  Value=ZERO_FLOAT
  Constant1 : Constant  Value=KVMC_CCAccelCMDUpLim_mps2
  Constant10 : Constant  Value=KVMC_GravityValue_mps2
  Constant11 : Constant  Value=KVMC_CCDevLowLim_mps2
  Constant12 : Constant  Value=ZERO_INT
  Constant19 : Constant  Value=KVMC_CCDevUpLim_mps2
  Constant2 : Constant  Value=KVMC_CCAccelCMDLowLim_mps2
  Constant3 : Constant  Value=KVMC_CCTqUpLim_Nm
  Constant4 : Constant  Value=KVMC_CCTqLowLim_Nm
  Constant5 : Constant  Value=KVMC_CCPedal2TqUpLim_Nm
  Constant6 : Constant  Value=KVMC_CCPedal2TqLowLim_Nm
  Constant7 : Constant  Value=KVMC_CCSpdDevUpLim_kph
  Constant8 : Constant  Value=KVMC_CCSpdDevLowLim_kph
  Constant9 : Constant  Value=KVMC_CCIGainOffDevSpd_kph
  Delay : Delay  DelayLength=1
  Detect Decrease : simulink/Logic and Bit Operations/Detect Decrease  vinit=0.0  OutDataTypeStr=boolean
  Detect Increase : simulink/Logic and Bit Operations/Detect Increase  vinit=0.0  OutDataTypeStr=boolean
  MVMC_CCDeltaTqIGain_Z_Nm : Lookup_n-D  BreakpointsForDimension1=AVMC_CCDeltaTqIGain_Y_mps2  BreakpointsForDimension2=AVMC_CCDeltaTqIGain_X_kph  Table=MVMC_CCDeltaTqIGain_Z_Nm  ExtrapMethod=Clip  InternalRulePriority=Speed  RndMeth=Simplest  InputSameDT=on
      settings: InputPortMap=u0,u1
  MVMC_CCDeltaTqPGain_Z_Nm : Lookup_n-D  BreakpointsForDimension1=AVMC_CCDeltaTqPGain_Y_kph  BreakpointsForDimension2=AVMC_CCDeltaTqPGain_X_kph  BreakpointsForDimension3=[5, 7]  Table=MVMC_CCDeltaTqPGain_Z_Nm  ExtrapMethod=Clip  InternalRulePriority=Speed  RndMeth=Simplest  InputSameDT=on
      settings: InputPortMap=u0,u1
  OR : Logic  Operator=OR  AllPortsSameDT=off  OutDataTypeStr=boolean
  Product : Product
  Relational Operator : RelationalOperator  Operator=<  OutDataTypeStr=boolean  RndMeth=Simplest
  Saturation Dynamic{,1..4} (5 alike) : simulink/Discontinuities/Saturation Dynamic  OutMin=[]  OutMax=[]  OutDataTypeStr=Inherit: Same as second input  OutDataType=fixdt(1, 16)  OutScaling=2^-10  DoSatur=off
  Switch : Switch  Criteria=u2 ~= 0
  Switch1 : Switch  Criteria=u2 ~= 0
  Switch2 : Switch  Criteria=u2 > Threshold
  Unit Delay : UnitDelay  SampleTime=-1  HasFrameUpgradeWarning=on
  VVMC_CruzWhlTqCal_Nm : Outport
  wires:
  Add4/1 -> Saturation Dynamic4/2
  Saturation Dynamic4/1 -> [VVMC_CCActSpdDev_kph], MVMC_CCDeltaTqPGain_Z_Nm/1  "VVMC_CCActSpdDev_kph"
  MVMC_CCDeltaTqPGain_Z_Nm/1 -> Add5/2  "VVMC_CCDeltaTqPGain_Nm"
  Add5/1 -> [VVMC_CCDeltaTq_Nm]  "VVMC_CCDeltaTq_Nm"
  [VVMC_CalMeterSpeed_kph] -> Add4/2
  Constant7/1 -> Saturation Dynamic4/1
  Constant8/1 -> Saturation Dynamic4/3
  Constant6/1 -> Saturation Dynamic/3
  Constant5/1 -> Saturation Dynamic/1
  Saturation Dynamic/1 -> Add1/1
  [VTQD_DriverWhlTqDem_Nm] -> Saturation Dynamic/2
  Delay/1 -> Detect Decrease/1
  Detect Increase/1 -> OR/1
  Detect Decrease/1 -> OR/2
  OR/1 -> Switch/2
  [VVMC_CruzActive_flg] -> Detect Increase/1
  [VVMC_CCPedalOvrd_flg] -> Delay/1
  Saturation Dynamic3/1 -> [VVMC_CruzWhlTqCal_Nm], Unit Delay/1  "VVMC_CruzWhlTqCal_Nm"
  VVMC_CCPedalOvrd_flg/1 -> [VVMC_CCPedalOvrd_flg]
  Switch1/1 -> Saturation Dynamic3/2
  Constant3/1 -> Saturation Dynamic3/1
  Constant4/1 -> Saturation Dynamic3/3
  Constant2/1 -> Saturation Dynamic2/3
  Constant1/1 -> Saturation Dynamic2/1
  CC Mode Acceleration Determination/1 -> Saturation Dynamic2/2
  Saturation Dynamic2/1 -> [VVMC_CCAccelCMD_mps2]  "VVMC_CCAccelCMD_mps2"
  VVMC_LongAcc_Gps/1 -> [VVMC_LongAcc_Gps]
  Product/1 -> Add3/2
  Saturation Dynamic1/1 -> MVMC_CCDeltaTqIGain_Z_Nm/1  "VVMC_ActCCAccDev_mps2"
  [VVMC_LongAcc_Gps] -> Product/1
  Add3/1 -> Saturation Dynamic1/2
  Constant10/1 -> Product/2
  [VVMC_CCAccelCMD_mps2] -> Add3/1
  Constant11/1 -> Saturation Dynamic1/3
  Constant19/1 -> Saturation Dynamic1/1
  [VVMC_CruzWhlTqCal_Nm] -> VVMC_CruzWhlTqCal_Nm/1
  VINP_VehSpeed_kph/1 -> [VINP_VehSpeed_kph]
  VVMC_CruzActive_flg/1 -> [VVMC_CruzActive_flg]
  VTQD_DriverWhlTqDem_Nm/1 -> [VTQD_DriverWhlTqDem_Nm]
  Unit Delay/1 -> [VVMC_LastCruzWhlTqCal_Nm]  "VVMC_LastCruzWhlTqCal_Nm"
  [VVMC_CruzActive_flg] -> Switch1/2
  [VVMC_CCDeltaTq_Nm] -> Add2/2
  [VVMC_LastCruzWhlTqCal_Nm] -> Add2/1
  [VVMC_CCDeltaTq_Nm] -> Add1/2
  [VINP_VehSpeed_kph] -> CC Mode Acceleration Determination/2
  VINP_SetSpd_kph/1 -> [VINP_SetSpd_kph]
  Constant/1 -> Switch1/3
  Switch/1 -> Switch1/1
  Add2/1 -> Switch/3
  Add1/1 -> Switch/1
  Add/1 -> CC Mode Acceleration Determination/1
  [VINP_VehSpeed_kph] -> MVMC_CCDeltaTqPGain_Z_Nm/2
  VVMC_CalMeterSpeed_kph/1 -> [VVMC_CalMeterSpeed_kph]
  [VVMC_CalMeterSpeed_kph] -> Add/2
  [VINP_VehSpeed_kph] -> MVMC_CCDeltaTqIGain_Z_Nm/2
  [VINP_SetSpd_kph] -> Add/1
  [VINP_SetSpd_kph] -> Add4/1
  Switch2/1 -> Add5/1  "VVMC_CCDeltaTqIGain_Nm"
  [VVMC_CCActSpdDev_kph] -> Abs/1
  Relational Operator/1 -> Switch2/2
  Constant12/1 -> Switch2/1
  Constant9/1 -> Relational Operator/2
  Abs/1 -> Relational Operator/1
  MVMC_CCDeltaTqIGain_Z_Nm/1 -> Switch2/3

== system vmc/VMC/CruiseControlFunction/CCTorqueSourceDetermination ==
  VTQD_DriverWhlTqDem_Nm : Inport
  VVMC_CruzWhlTqCal_Nm : Inport  Port=2
  VVMC_CruzActive_flg : Inport  Port=3
  VTQD_LowIdleAccPedal_flg : Inport  Port=4
  AND : Logic  Inputs=3  AllPortsSameDT=off  OutDataTypeStr=boolean
  Constant1 : Constant  Value=FALSE
  Constant3 : Constant  Value=TRUE
  NOT : Logic  Operator=NOT  AllPortsSameDT=off  OutDataTypeStr=boolean
  Relational Operator : RelationalOperator  OutDataTypeStr=boolean  RndMeth=Simplest
  Switch : Switch  Criteria=u2 ~= 0
  Switch1 : Switch  Criteria=u2 ~= 0
  VVMC_CruzWhlTqReq_Nm : Outport
  VVMC_CCPedalOvrd_flg : Outport  Port=2
  wires:
  [VVMC_CCPedalOvrd_flg] -> VVMC_CCPedalOvrd_flg/1
  Switch1/1 -> [VVMC_CCPedalOvrd_flg]  "VVMC_CCPedalOvrd_flg"
  Constant1/1 -> Switch1/3
  Constant3/1 -> Switch1/1
  NOT/1 -> AND/3
  [VTQD_LowIdleAccPedal_flg] -> NOT/1
  [VVMC_CruzActive_flg] -> AND/1
  AND/1 -> Switch/2, Switch1/2
  Relational Operator/1 -> AND/2
  VTQD_LowIdleAccPedal_flg/1 -> [VTQD_LowIdleAccPedal_flg]
  VVMC_CruzActive_flg/1 -> [VVMC_CruzActive_flg]
  [VVMC_CruzWhlTqReq_Nm] -> VVMC_CruzWhlTqReq_Nm/1
  VVMC_CruzWhlTqCal_Nm/1 -> [VVMC_CruzWhlTqCal_Nm]
  VTQD_DriverWhlTqDem_Nm/1 -> [VTQD_DriverWhlTqDem_Nm]
  [VTQD_DriverWhlTqDem_Nm] -> Relational Operator/1
  Switch/1 -> [VVMC_CruzWhlTqReq_Nm]  "VVMC_CruzWhlTqReq_Nm"
  [VVMC_CruzWhlTqCal_Nm] -> Relational Operator/2
  [VTQD_DriverWhlTqDem_Nm] -> Switch/1
  [VVMC_CruzWhlTqCal_Nm] -> Switch/3

== system vmc/VMC/IMU/IMU memorized offset result ==
  VINP_MemOffsetGyroX_raw16 : Inport
  VINP_MemOffsetGyroY_raw16 : Inport  Port=2
  VINP_MemOffsetGyroZ_raw16 : Inport  Port=3
  VINP_MemOffsetAccX_raw16 : Inport  Port=4
  VINP_MemOffsetAccY_raw16 : Inport  Port=5
  VINP_MemOffsetAccZ_raw16 : Inport  Port=6
  ACCEL_FS_SEL = 001 SENSITIVITY = 2000 LSB/g : Constant  Value=KVMC_AccFSCalSet_enum
  Constant6 : Constant  Value=ONE_FLOAT  OutDataTypeStr=single
  Data Type Conversion : DataTypeConversion  OutDataTypeStr=uint16
  Data Type Conversion{1..6} (6 alike) : DataTypeConversion  OutDataTypeStr=single
  Data Type Conversion7 : DataTypeConversion  OutDataTypeStr=uint16
  Divide{,1..5} (6 alike) : Product  Inputs=**
  GYRO_FS_SEL = 0001 SENSITIVITY = 50 LSB/dps : Constant  Value=KVMC_GyroFSCalSet_enum
  Math Function{,1..5} (6 alike) : Math  Operator=reciprocal  SaturateOnIntegerOverflow=on
  Plus : Sum  Inputs=+-
  VVMC_MemOffsetGyroX_Dps : Outport
  VVMC_MemOffsetGyroY_Dps : Outport  Port=2
  VVMC_MemOffsetGyroZ_Dps : Outport  Port=3
  VVMC_MemOffsetAccX_G : Outport  Port=4
  VVMC_MemOffsetAccY_G : Outport  Port=5
  VVMC_MemOffsetAccZ_G : Outport  Port=6
  wires:
  VINP_MemOffsetGyroX_raw16/1 -> [VINP_MemOffsetGyroX_raw16]
  VINP_MemOffsetGyroY_raw16/1 -> [VINP_MemOffsetGyroY_raw16]
  [VINP_MemOffsetGyroX_raw16] -> Divide/1
  [VVMC_GyroFSCalSet_enum] -> Data Type Conversion1/1
  GYRO_FS_SEL = 0001 SENSITIVITY = 50 LSB/dps/1 -> Data Type Conversion/1
  Data Type Conversion/1 -> [VVMC_GyroFSCalSet_enum]  "VVMC_GyroFSCalSet_enum"
  [VVMC_GyroFSCalSet_enum] -> Data Type Conversion2/1
  [VINP_MemOffsetGyroY_raw16] -> Divide1/1
  [VINP_MemOffsetGyroZ_raw16] -> Divide2/1
  [VVMC_GyroFSCalSet_enum] -> Data Type Conversion3/1
  [VVMC_AccFSCalSet_enum] -> Data Type Conversion4/1
  [VINP_MemOffsetAccX_raw16] -> Divide3/1
  [VINP_MemOffsetAccY_raw16] -> Divide4/1
  [VVMC_AccFSCalSet_enum] -> Data Type Conversion5/1
  [VVMC_AccFSCalSet_enum] -> Data Type Conversion6/1
  [VINP_MemOffsetAccZ_raw16] -> Divide5/1
  Data Type Conversion7/1 -> [VVMC_AccFSCalSet_enum]  "VVMC_AccFSCalSet_enum"
  ACCEL_FS_SEL = 001 SENSITIVITY = 2000 LSB/g/1 -> Data Type Conversion7/1
  Divide/1 -> [VVMC_MemOffsetGyroX_Dps]  "VVMC_MemOffsetGyroX_Dps"
  Divide1/1 -> [VVMC_MemOffsetGyroY_Dps]  "VVMC_MemOffsetGyroY_Dps"
  Divide2/1 -> [VVMC_MemOffsetGyroZ_Dps]  "VVMC_MemOffsetGyroZ_Dps"
  Divide3/1 -> [VVMC_MemOffsetAccX_G]  "VVMC_MemOffsetAccX_G"
  Plus/1 -> [VVMC_MemOffsetAccZ_G]  "VVMC_MemOffsetAccZ_G"
  Divide5/1 -> Plus/1
  Constant6/1 -> Plus/2
  [VVMC_MemOffsetGyroX_Dps] -> VVMC_MemOffsetGyroX_Dps/1
  [VVMC_MemOffsetGyroY_Dps] -> VVMC_MemOffsetGyroY_Dps/1
  [VVMC_MemOffsetGyroZ_Dps] -> VVMC_MemOffsetGyroZ_Dps/1
  [VVMC_MemOffsetAccX_G] -> VVMC_MemOffsetAccX_G/1
  [VVMC_MemOffsetAccY_G] -> VVMC_MemOffsetAccY_G/1
  [VVMC_MemOffsetAccZ_G] -> VVMC_MemOffsetAccZ_G/1
  Divide4/1 -> [VVMC_MemOffsetAccY_G]  "VVMC_MemOffsetAccY_G"
  VINP_MemOffsetGyroZ_raw16/1 -> [VINP_MemOffsetGyroZ_raw16]
  VINP_MemOffsetAccX_raw16/1 -> [VINP_MemOffsetAccX_raw16]
  VINP_MemOffsetAccY_raw16/1 -> [VINP_MemOffsetAccY_raw16]
  VINP_MemOffsetAccZ_raw16/1 -> [VINP_MemOffsetAccZ_raw16]
  Math Function/1 -> Divide/2
  Math Function1/1 -> Divide1/2
  Math Function2/1 -> Divide2/2
  Math Function3/1 -> Divide3/2
  Math Function4/1 -> Divide4/2
  Math Function5/1 -> Divide5/2
  Data Type Conversion1/1 -> Math Function/1
  Data Type Conversion2/1 -> Math Function1/1
  Data Type Conversion3/1 -> Math Function2/1
  Data Type Conversion4/1 -> Math Function3/1
  Data Type Conversion5/1 -> Math Function4/1
  Data Type Conversion6/1 -> Math Function5/1
